simulink model "embedded_with_return"  (Simulink 7.6)
settings: Solver=FixedStepDiscrete  StartTime=0.0  StopTime=10.0  FixedStep=1  RelTol=1e-3
settings Model: Creator=Harmon S. Nine  LastModifiedBy=c2wt
settings DebuggingCC: StrictBusMsg=Warning
settings SFSimCC: SimParseCustomCode=off

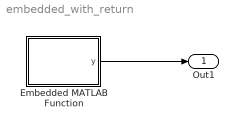
== system embedded_with_return ==
  Embedded MATLAB Function : Stateflow chart  TreatAsAtomicUnit=on
  Out1 : Outport
  wires:
  Embedded MATLAB Function/1(y) -> Out1/1

== matlab function Embedded MATLAB Function ==
  data: y output double
function y = fcn()
%#eml

temp = 1
if temp == 1
    y = 1
    return
end

y = 2
